simulink model "MDR_AA_TMD_Intercepteur"  (R2019b)
settings: Solver=ode4  StartTime=0.0  StopTime=Inf  FixedStep=0.01  RelTol=1e-3
values from neighbouring files (symbols this model uses):
  stdatm = [0 100 200 300 400 500 600 700 800 900 1000 1100 ... (4305 elements, 861x5)]    [stdatm.mat]
undefined symbols (not defined in the file or in its folder): Aero_Struct_CM, Aero_TMD, e0_0, e1_0, e2_0, e3_0, magnitude, Masse_Inertie_TMD, pow, Propu_TMD, Simu_TMD, Vm_0, xme_0
libraries: simulink x17
(part 4 of 4)

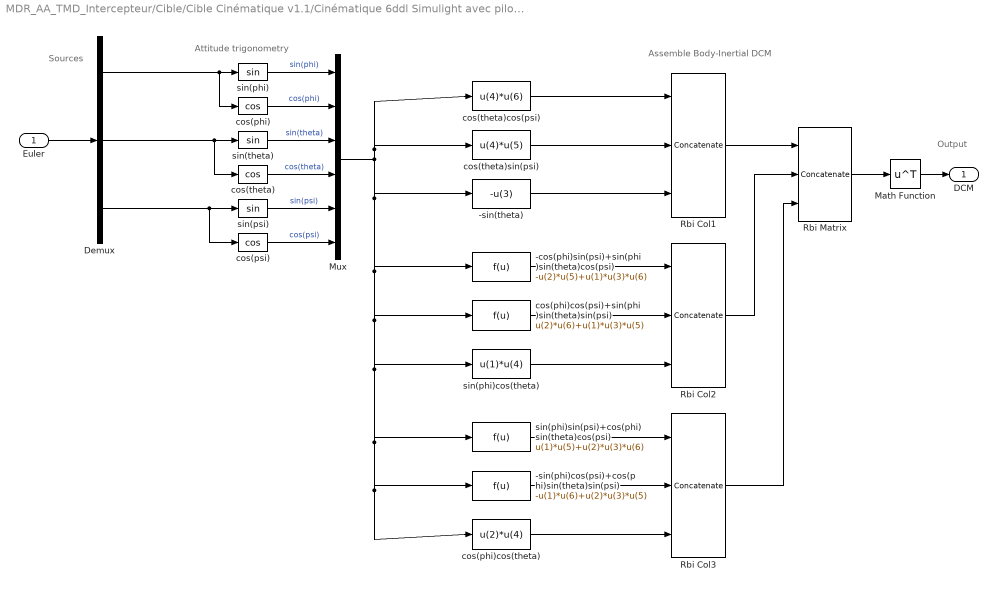
== system MDR_AA_TMD_Intercepteur/Cible/Cible Cinématique v1.1/Cinématique 6ddl Simulight avec pilotage en force/Pesanteur/Inert2Miss/Euler2DCM ==
  note: Attitude trigonometry
  note: Sources
  note: Output
  note: Assemble Body-Inertial DCM
  Euler : Inport  PortDimensions=[3 1]
  -cos(phi)sin(psi)+sin(phi)sin(theta)cos(psi) : Fcn  Expr=-u(2)*u(5)+u(1)*u(3)*u(6)
  -sin(phi)cos(psi)+cos(phi)sin(theta)sin(psi) : Fcn  Expr=-u(1)*u(6)+u(2)*u(3)*u(5)
  -sin(theta) : Fcn  Expr=-u(3)
  Demux : Demux  Outputs=3
  Math Function : Math  Operator=transpose  SaturateOnIntegerOverflow=on
  Mux : Mux  Inputs=6
  Rbi Matrix : Concatenate  NumInputs=3  Mode=Multidimensional array  ConcatenateDimension=2
  Rbi Col1 : Concatenate  NumInputs=3  Mode=Multidimensional array
  Rbi Col2 : Concatenate  NumInputs=3  Mode=Multidimensional array
  Rbi Col3 : Concatenate  NumInputs=3  Mode=Multidimensional array
  cos(phi) : Trigonometry  Operator=cos
  cos(phi)cos(psi)+sin(phi)sin(theta)sin(psi) : Fcn  Expr=u(2)*u(6)+u(1)*u(3)*u(5)
  cos(phi)cos(theta) : Fcn  Expr=u(2)*u(4)
  cos(psi) : Trigonometry  Operator=cos
  cos(theta) : Trigonometry  Operator=cos
  cos(theta)cos(psi) : Fcn  Expr=u(4)*u(6)
  cos(theta)sin(psi) : Fcn  Expr=u(4)*u(5)
  sin(phi) : Trigonometry
  sin(phi)cos(theta) : Fcn  Expr=u(1)*u(4)
  sin(phi)sin(psi)+cos(phi)sin(theta)cos(psi) : Fcn  Expr=u(1)*u(5)+u(2)*u(3)*u(6)
  sin(psi) : Trigonometry
  sin(theta) : Trigonometry
  DCM : Outport  VectorParamsAs1DForOutWhenUnconnected=off
  wires:
  Demux/3 -> sin(psi)/1, cos(psi)/1
  Demux/2 -> sin(theta)/1, cos(theta)/1
  Demux/1 -> cos(phi)/1, sin(phi)/1
  Euler/1 -> Demux/1
  sin(phi)/1 -> Mux/1  "sin(phi)"
  cos(phi)/1 -> Mux/2  "cos(phi)"
  sin(theta)/1 -> Mux/3  "sin(theta)"
  cos(theta)/1 -> Mux/4  "cos(theta)"
  sin(psi)/1 -> Mux/5  "sin(psi)"
  cos(psi)/1 -> Mux/6  "cos(psi)"
  Mux/1 -> cos(theta)cos(psi)/1, cos(theta)sin(psi)/1, sin(phi)sin(psi)+cos(phi)sin(theta)cos(psi)/1, cos(phi)cos(theta)/1, -sin(phi)cos(psi)+cos(phi)sin(theta)sin(psi)/1, sin(phi)cos(theta)/1, cos(phi)cos(psi)+sin(phi)sin(theta)sin(psi)/1, -cos(phi)sin(psi)+sin(phi)sin(theta)cos(psi)/1, -sin(theta)/1
  Math Function/1 -> DCM/1
  Rbi Matrix/1 -> Math Function/1
  Rbi Col1/1 -> Rbi Matrix/1
  cos(theta)cos(psi)/1 -> Rbi Col1/1
  cos(theta)sin(psi)/1 -> Rbi Col1/2
  -sin(theta)/1 -> Rbi Col1/3
  -cos(phi)sin(psi)+sin(phi)sin(theta)cos(psi)/1 -> Rbi Col2/1
  cos(phi)cos(psi)+sin(phi)sin(theta)sin(psi)/1 -> Rbi Col2/2
  sin(phi)cos(theta)/1 -> Rbi Col2/3
  sin(phi)sin(psi)+cos(phi)sin(theta)cos(psi)/1 -> Rbi Col3/1
  -sin(phi)cos(psi)+cos(phi)sin(theta)sin(psi)/1 -> Rbi Col3/2
  cos(phi)cos(theta)/1 -> Rbi Col3/3
  Rbi Col2/1 -> Rbi Matrix/2
  Rbi Col3/1 -> Rbi Matrix/3

== system MDR_AA_TMD_Intercepteur/Cible/Cible Cinématique v1.1/Pilote 2 axes Simulight à partir de gradient/Alpha commandé - Plan de tangage/Zero Offset/Non-zero Sign ==
  In : Inport
  One : Constant
  Relational Operator : RelationalOperator  Operator===  RndMeth=Nearest  InputSameDT=on
  Sign : Signum
  Switch : Switch  Threshold=1  SaturateOnIntegerOverflow=on  InputSameDT=on
  Zero : Constant  Value=0
  Out : Outport  VectorParamsAs1DForOutWhenUnconnected=off
  wires:
  Switch/1 -> Out/1
  Sign/1 -> Switch/3
  One/1 -> Switch/1
  Relational Operator/1 -> Switch/2
  In/1 -> Sign/1, Relational Operator/1
  Zero/1 -> Relational Operator/2

== system MDR_AA_TMD_Intercepteur/Cible/Cible Cinématique v1.1/Pilote 2 axes Simulight à partir de gradient/Beta commandé - Plan de lacet/Zero Offset/Non-zero Sign ==
  In : Inport
  One : Constant
  Relational Operator : RelationalOperator  Operator===  RndMeth=Nearest  InputSameDT=on
  Sign : Signum
  Switch : Switch  Threshold=1  SaturateOnIntegerOverflow=on  InputSameDT=on
  Zero : Constant  Value=0
  Out : Outport  VectorParamsAs1DForOutWhenUnconnected=off
  wires:
  Zero/1 -> Relational Operator/2
  In/1 -> Relational Operator/1, Sign/1
  Relational Operator/1 -> Switch/2
  One/1 -> Switch/1
  Sign/1 -> Switch/3
  Switch/1 -> Out/1

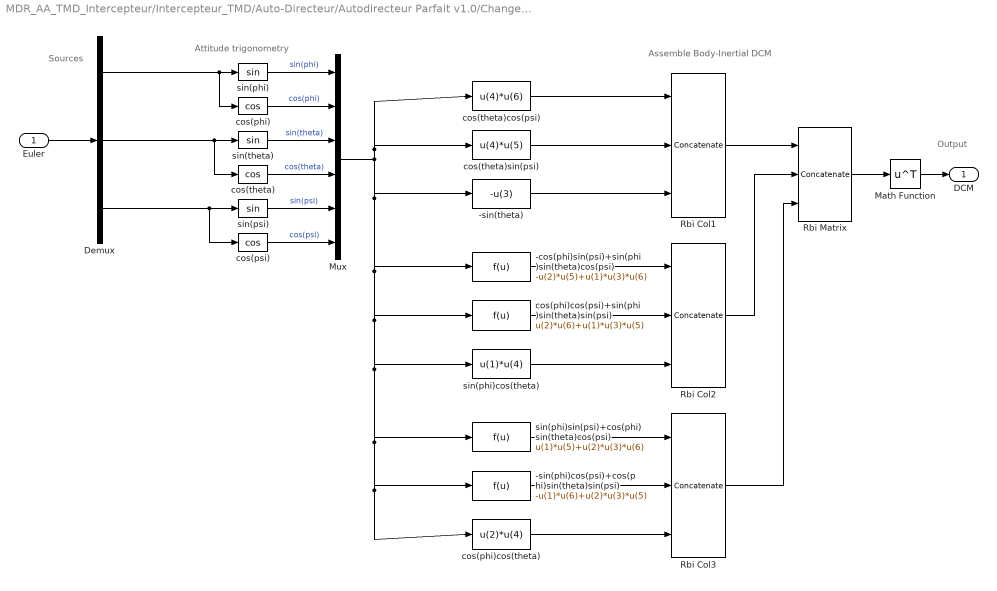
== system MDR_AA_TMD_Intercepteur/Intercepteur_TMD/Auto-Directeur/Autodirecteur Parfait v1.0/Changement de repère inertiel -> miss/Inert2Miss1/Euler2DCM ==
  note: Attitude trigonometry
  note: Sources
  note: Output
  note: Assemble Body-Inertial DCM
  Euler : Inport  PortDimensions=[3 1]
  -cos(phi)sin(psi)+sin(phi)sin(theta)cos(psi) : Fcn  Expr=-u(2)*u(5)+u(1)*u(3)*u(6)
  -sin(phi)cos(psi)+cos(phi)sin(theta)sin(psi) : Fcn  Expr=-u(1)*u(6)+u(2)*u(3)*u(5)
  -sin(theta) : Fcn  Expr=-u(3)
  Demux : Demux  Outputs=3
  Math Function : Math  Operator=transpose  SaturateOnIntegerOverflow=on
  Mux : Mux  Inputs=6
  Rbi Matrix : Concatenate  NumInputs=3  Mode=Multidimensional array  ConcatenateDimension=2
  Rbi Col1 : Concatenate  NumInputs=3  Mode=Multidimensional array
  Rbi Col2 : Concatenate  NumInputs=3  Mode=Multidimensional array
  Rbi Col3 : Concatenate  NumInputs=3  Mode=Multidimensional array
  cos(phi) : Trigonometry  Operator=cos
  cos(phi)cos(psi)+sin(phi)sin(theta)sin(psi) : Fcn  Expr=u(2)*u(6)+u(1)*u(3)*u(5)
  cos(phi)cos(theta) : Fcn  Expr=u(2)*u(4)
  cos(psi) : Trigonometry  Operator=cos
  cos(theta) : Trigonometry  Operator=cos
  cos(theta)cos(psi) : Fcn  Expr=u(4)*u(6)
  cos(theta)sin(psi) : Fcn  Expr=u(4)*u(5)
  sin(phi) : Trigonometry
  sin(phi)cos(theta) : Fcn  Expr=u(1)*u(4)
  sin(phi)sin(psi)+cos(phi)sin(theta)cos(psi) : Fcn  Expr=u(1)*u(5)+u(2)*u(3)*u(6)
  sin(psi) : Trigonometry
  sin(theta) : Trigonometry
  DCM : Outport  VectorParamsAs1DForOutWhenUnconnected=off
  wires:
  Demux/3 -> sin(psi)/1, cos(psi)/1
  Demux/2 -> sin(theta)/1, cos(theta)/1
  Demux/1 -> cos(phi)/1, sin(phi)/1
  Euler/1 -> Demux/1
  sin(phi)/1 -> Mux/1  "sin(phi)"
  cos(phi)/1 -> Mux/2  "cos(phi)"
  sin(theta)/1 -> Mux/3  "sin(theta)"
  cos(theta)/1 -> Mux/4  "cos(theta)"
  sin(psi)/1 -> Mux/5  "sin(psi)"
  cos(psi)/1 -> Mux/6  "cos(psi)"
  Mux/1 -> cos(theta)cos(psi)/1, cos(theta)sin(psi)/1, sin(phi)sin(psi)+cos(phi)sin(theta)cos(psi)/1, cos(phi)cos(theta)/1, -sin(phi)cos(psi)+cos(phi)sin(theta)sin(psi)/1, sin(phi)cos(theta)/1, cos(phi)cos(psi)+sin(phi)sin(theta)sin(psi)/1, -cos(phi)sin(psi)+sin(phi)sin(theta)cos(psi)/1, -sin(theta)/1
  Math Function/1 -> DCM/1
  Rbi Matrix/1 -> Math Function/1
  Rbi Col1/1 -> Rbi Matrix/1
  cos(theta)cos(psi)/1 -> Rbi Col1/1
  cos(theta)sin(psi)/1 -> Rbi Col1/2
  -sin(theta)/1 -> Rbi Col1/3
  -cos(phi)sin(psi)+sin(phi)sin(theta)cos(psi)/1 -> Rbi Col2/1
  cos(phi)cos(psi)+sin(phi)sin(theta)sin(psi)/1 -> Rbi Col2/2
  sin(phi)cos(theta)/1 -> Rbi Col2/3
  sin(phi)sin(psi)+cos(phi)sin(theta)cos(psi)/1 -> Rbi Col3/1
  -sin(phi)cos(psi)+cos(phi)sin(theta)sin(psi)/1 -> Rbi Col3/2
  cos(phi)cos(theta)/1 -> Rbi Col3/3
  Rbi Col2/1 -> Rbi Matrix/2
  Rbi Col3/1 -> Rbi Matrix/3

== system MDR_AA_TMD_Intercepteur/Intercepteur_TMD/Bloc Cinématique/Cinématique 6ddl Simulight avec pilotage en force/Calcul des pqr/pqr_a/dérive alpha//beta ==
  AlphaR : Inport
  BetaR : Inport  Port=2
  Clock : Clock
  Divide : Product  Inputs=*/
  Divide1 : Product  Inputs=*/
  IC : InitialCondition
  Memory : Memory
  Memory1 : Memory
  Memory2 : Memory
  Sum : Sum  Inputs=|+-
  Sum1 : Sum  Inputs=|+-
  Sum2 : Sum  Inputs=|+-
  dAlphaR : Outport  VectorParamsAs1DForOutWhenUnconnected=off
  dBetaR : Outport  Port=2  VectorParamsAs1DForOutWhenUnconnected=off
  wires:
  AlphaR/1 -> Memory/1, Sum/1
  Memory/1 -> Sum/2
  Sum/1 -> Divide/1
  BetaR/1 -> Sum1/1, Memory1/1
  Memory1/1 -> Sum1/2
  Sum1/1 -> Divide1/1
  Divide/1 -> dAlphaR/1
  Divide1/1 -> dBetaR/1
  Clock/1 -> Memory2/1, Sum2/1
  Memory2/1 -> Sum2/2
  Sum2/1 -> IC/1
  IC/1 -> Divide1/2, Divide/2

== system MDR_AA_TMD_Intercepteur/Intercepteur_TMD/Bloc Cinématique/Cinématique 6ddl Simulight avec pilotage en force/Equations des forces/Gestion de sortie de rampe/Norme ==
  V : Inport
  Dot Product : DotProduct  InputSameDT=on  OutDataTypeStr=Inherit: Inherit via internal rule
  Sqrt : Math  Operator=sqrt  SaturateOnIntegerOverflow=on
  ||V|| : Outport  VectorParamsAs1DForOutWhenUnconnected=off
  wires:
  Sqrt/1 -> ||V||/1
  V/1 -> Dot Product/2, Dot Product/1
  Dot Product/1 -> Sqrt/1

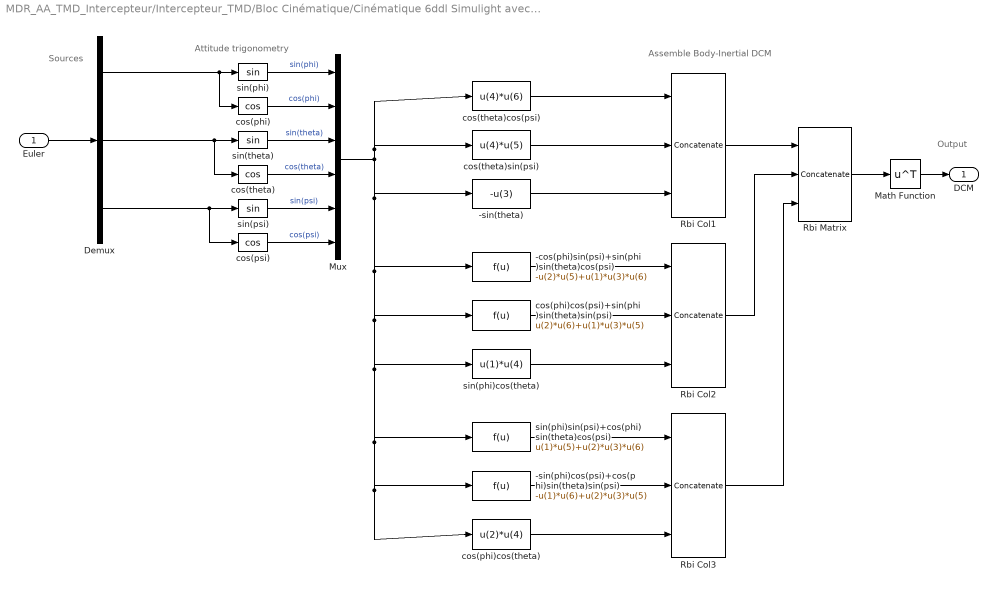
== system MDR_AA_TMD_Intercepteur/Intercepteur_TMD/Bloc Cinématique/Cinématique 6ddl Simulight avec pilotage en force/Pesanteur/Inert2Miss/Euler2DCM ==
  note: Attitude trigonometry
  note: Sources
  note: Output
  note: Assemble Body-Inertial DCM
  Euler : Inport  PortDimensions=[3 1]
  -cos(phi)sin(psi)+sin(phi)sin(theta)cos(psi) : Fcn  Expr=-u(2)*u(5)+u(1)*u(3)*u(6)
  -sin(phi)cos(psi)+cos(phi)sin(theta)sin(psi) : Fcn  Expr=-u(1)*u(6)+u(2)*u(3)*u(5)
  -sin(theta) : Fcn  Expr=-u(3)
  Demux : Demux  Outputs=3
  Math Function : Math  Operator=transpose  SaturateOnIntegerOverflow=on
  Mux : Mux  Inputs=6
  Rbi Matrix : Concatenate  NumInputs=3  Mode=Multidimensional array  ConcatenateDimension=2
  Rbi Col1 : Concatenate  NumInputs=3  Mode=Multidimensional array
  Rbi Col2 : Concatenate  NumInputs=3  Mode=Multidimensional array
  Rbi Col3 : Concatenate  NumInputs=3  Mode=Multidimensional array
  cos(phi) : Trigonometry  Operator=cos
  cos(phi)cos(psi)+sin(phi)sin(theta)sin(psi) : Fcn  Expr=u(2)*u(6)+u(1)*u(3)*u(5)
  cos(phi)cos(theta) : Fcn  Expr=u(2)*u(4)
  cos(psi) : Trigonometry  Operator=cos
  cos(theta) : Trigonometry  Operator=cos
  cos(theta)cos(psi) : Fcn  Expr=u(4)*u(6)
  cos(theta)sin(psi) : Fcn  Expr=u(4)*u(5)
  sin(phi) : Trigonometry
  sin(phi)cos(theta) : Fcn  Expr=u(1)*u(4)
  sin(phi)sin(psi)+cos(phi)sin(theta)cos(psi) : Fcn  Expr=u(1)*u(5)+u(2)*u(3)*u(6)
  sin(psi) : Trigonometry
  sin(theta) : Trigonometry
  DCM : Outport  VectorParamsAs1DForOutWhenUnconnected=off
  wires:
  Demux/3 -> sin(psi)/1, cos(psi)/1
  Demux/2 -> sin(theta)/1, cos(theta)/1
  Demux/1 -> cos(phi)/1, sin(phi)/1
  Euler/1 -> Demux/1
  sin(phi)/1 -> Mux/1  "sin(phi)"
  cos(phi)/1 -> Mux/2  "cos(phi)"
  sin(theta)/1 -> Mux/3  "sin(theta)"
  cos(theta)/1 -> Mux/4  "cos(theta)"
  sin(psi)/1 -> Mux/5  "sin(psi)"
  cos(psi)/1 -> Mux/6  "cos(psi)"
  Mux/1 -> cos(theta)cos(psi)/1, cos(theta)sin(psi)/1, sin(phi)sin(psi)+cos(phi)sin(theta)cos(psi)/1, cos(phi)cos(theta)/1, -sin(phi)cos(psi)+cos(phi)sin(theta)sin(psi)/1, sin(phi)cos(theta)/1, cos(phi)cos(psi)+sin(phi)sin(theta)sin(psi)/1, -cos(phi)sin(psi)+sin(phi)sin(theta)cos(psi)/1, -sin(theta)/1
  Math Function/1 -> DCM/1
  Rbi Matrix/1 -> Math Function/1
  Rbi Col1/1 -> Rbi Matrix/1
  cos(theta)cos(psi)/1 -> Rbi Col1/1
  cos(theta)sin(psi)/1 -> Rbi Col1/2
  -sin(theta)/1 -> Rbi Col1/3
  -cos(phi)sin(psi)+sin(phi)sin(theta)cos(psi)/1 -> Rbi Col2/1
  cos(phi)cos(psi)+sin(phi)sin(theta)sin(psi)/1 -> Rbi Col2/2
  sin(phi)cos(theta)/1 -> Rbi Col2/3
  sin(phi)sin(psi)+cos(phi)sin(theta)cos(psi)/1 -> Rbi Col3/1
  -sin(phi)cos(psi)+cos(phi)sin(theta)sin(psi)/1 -> Rbi Col3/2
  cos(phi)cos(theta)/1 -> Rbi Col3/3
  Rbi Col2/1 -> Rbi Matrix/2
  Rbi Col3/1 -> Rbi Matrix/3

== system MDR_AA_TMD_Intercepteur/Intercepteur_TMD/Calculateur/Pilotage/Pilote 2 axes Simulight avec prise en compte de la manoeuvrabilité max/Alpha commandé - Plan de tangage/Calcul de CN0 ==
  Alpha : Inport
  Mach : Inport  Port=2
  CN_0 : Lookup_n-D  BreakpointsForDimension1=vAlpha  BreakpointsForDimension2=vMach  BreakpointsForDimension3=Aero_Struct_CM.vBrq  Table=CN  ExtrapMethod=Clip  UseLastTableValue=on  RndMeth=Simplest  InputSameDT=on
  vCN0 : Outport  VectorParamsAs1DForOutWhenUnconnected=off
  wires:
  CN_0/1 -> vCN0/1
  Mach/1 -> CN_0/2
  Alpha/1 -> CN_0/1

== system MDR_AA_TMD_Intercepteur/Intercepteur_TMD/Calculateur/Pilotage/Pilote 2 axes Simulight avec prise en compte de la manoeuvrabilité max/Alpha commandé - Plan de tangage/Calcul du coefficient de CN commandé avec gestion de la division par 0 ==
  GcoV : Inport
  Masse : Inport  Port=2
  Pression_dynamique : Inport  Port=3
  Compare To Zero : simulink/Logic and Bit Operations/Compare To Zero  relop===  OutDataTypeStr=boolean  ZeroCross=off
  Divide1 : Product  Inputs=*/
  Memory : Memory
  Product : Product  RndMeth=Zero
  Switch : Switch  Criteria=u2 > Threshold
  Zero Offset : Subsystem  mask(Zero offset){tol=10^-6}
      mask prompts: tol "Tolerance"
      mask help: This block outputs a value equal to the tolerance specified in the block parameters if the input falls within a sphere with this tolerance as radius and center in the origin. Otherwise, the output equals the input.
      mask Help: eval('OpenHelp(''A3_Blockset.mdl'', ''..\Help\Toolbox\Tools\Zero_offset.html'')');
  CN_co : Outport  VectorParamsAs1DForOutWhenUnconnected=off
  wires:
  Pression_dynamique/1 -> Compare To Zero/1, Zero Offset/1(In)
  Switch/1 -> CN_co/1, Memory/1
  Compare To Zero/1 -> Switch/2
  GcoV/1 -> Product/2
  Masse/1 -> Divide1/1
  Divide1/1 -> Product/1
  Product/1 -> Switch/3
  Memory/1 -> Switch/1
  Zero Offset/1(Out) -> Divide1/2

== system MDR_AA_TMD_Intercepteur/Intercepteur_TMD/Calculateur/Pilotage/Pilote 2 axes Simulight avec prise en compte de la manoeuvrabilité max/Alpha commandé - Plan de tangage/Interpolation linéaire pour trouver l'incidence correspondant au coefficient de portance commandé ==
  CN_co_sat : Inport
  vCN0 : Inport  Port=2
  vAlpha : Inport  Port=3
  Lookup Table Dynamic : simulink/Lookup Tables/Lookup Table Dynamic  LookUpMeth=Interpolation-Use End Values  OutDataType=fixdt('double')  OutScaling=[]  OutputDataTypeScalingMode=Specify via dialog  OutDataTypeStr=fixdt('double')  DoSatur=off
      settings: SourceProductName=Simulink
  deg2rad : Gain  Gain=pi/180
  Alphaco : Outport  VectorParamsAs1DForOutWhenUnconnected=off
  wires:
  deg2rad/1 -> Alphaco/1
  vCN0/1 -> Lookup Table Dynamic/2
  CN_co_sat/1 -> Lookup Table Dynamic/1
  vAlpha/1 -> Lookup Table Dynamic/3
  Lookup Table Dynamic/1 -> deg2rad/1

== system MDR_AA_TMD_Intercepteur/Intercepteur_TMD/Calculateur/Pilotage/Pilote 2 axes Simulight avec prise en compte de la manoeuvrabilité max/Alpha commandé - Plan de tangage/Saturation de CN_co par la valeur max de CN équilibré ==
  Mach : Inport
  CN_co : Inport  Port=2
  CNmax : Lookup_n-D  NumberOfTableDimensions=1  BreakpointsForDimension1=vMach_CNmax  Table=CNmax  ExtrapMethod=Clip  UseLastTableValue=on  RndMeth=Simplest  InputSameDT=on
  Gain : Gain  Gain=-1
  Saturation Dynamic : simulink/Discontinuities/Saturation Dynamic  OutMin=[]  OutMax=[]  OutDataTypeStr=Inherit: Same as second input  OutDataType=fixdt(1, 16)  OutScaling=2^-10  DoSatur=off
  CN_co_sat : Outport  VectorParamsAs1DForOutWhenUnconnected=off
  wires:
  Saturation Dynamic/1 -> CN_co_sat/1
  CN_co/1 -> Saturation Dynamic/2
  Mach/1 -> CNmax/1
  Gain/1 -> Saturation Dynamic/3
  CNmax/1 -> Gain/1, Saturation Dynamic/1

== system MDR_AA_TMD_Intercepteur/Intercepteur_TMD/Calculateur/Pilotage/Pilote 2 axes Simulight avec prise en compte de la manoeuvrabilité max/Beta commandé - Plan de lacet/Calcul de CY0 ==
  Beta : Inport
  Mach : Inport  Port=2
  CY_0 : Lookup_n-D  BreakpointsForDimension1=vBeta  BreakpointsForDimension2=vMach  BreakpointsForDimension3=Aero_Struct_CM.vBrq  Table=CY  ExtrapMethod=Clip  UseLastTableValue=on  RndMeth=Simplest  InputSameDT=on
  vCY0 : Outport  VectorParamsAs1DForOutWhenUnconnected=off
  wires:
  Beta/1 -> CY_0/1
  Mach/1 -> CY_0/2
  CY_0/1 -> vCY0/1

== system MDR_AA_TMD_Intercepteur/Intercepteur_TMD/Calculateur/Pilotage/Pilote 2 axes Simulight avec prise en compte de la manoeuvrabilité max/Beta commandé - Plan de lacet/Calcul du coefficient de CY commandé avec gestion de la division par 0 ==
  GcoH : Inport
  Masse : Inport  Port=2
  Pression_dynamique : Inport  Port=3
  Compare To Zero : simulink/Logic and Bit Operations/Compare To Zero  relop===  OutDataTypeStr=boolean  ZeroCross=off
  Divide1 : Product  Inputs=*/
  Memory : Memory
  Product : Product  RndMeth=Zero
  Switch : Switch  Criteria=u2 > Threshold
  Zero Offset : Subsystem  mask(Zero offset){tol=10^-6}
      mask prompts: tol "Tolerance"
      mask help: This block outputs a value equal to the tolerance specified in the block parameters if the input falls within a sphere with this tolerance as radius and center in the origin. Otherwise, the output equals the input.
      mask Help: eval('OpenHelp(''A3_Blockset.mdl'', ''..\Help\Toolbox\Tools\Zero_offset.html'')');
  CY_co : Outport  VectorParamsAs1DForOutWhenUnconnected=off
  wires:
  Pression_dynamique/1 -> Compare To Zero/1, Zero Offset/1(In)
  Switch/1 -> CY_co/1, Memory/1
  Compare To Zero/1 -> Switch/2
  GcoH/1 -> Product/2
  Masse/1 -> Divide1/1
  Divide1/1 -> Product/1
  Product/1 -> Switch/3
  Memory/1 -> Switch/1
  Zero Offset/1(Out) -> Divide1/2

== system MDR_AA_TMD_Intercepteur/Intercepteur_TMD/Calculateur/Pilotage/Pilote 2 axes Simulight avec prise en compte de la manoeuvrabilité max/Beta commandé - Plan de lacet/Interpolation linéaire pour trouver le dérapage correspondant au coefficient de portance commandé ==
  CY_co_sat : Inport
  vCY0 : Inport  Port=2
  vBeta : Inport  Port=3
  Lookup Table Dynamic : simulink/Lookup Tables/Lookup Table Dynamic  LookUpMeth=Interpolation-Use End Values  OutDataType=fixdt('double')  OutScaling=[]  OutputDataTypeScalingMode=Specify via dialog  OutDataTypeStr=fixdt('double')  DoSatur=off
      settings: SourceProductName=Simulink
  deg2rad : Gain  Gain=pi/180
  Betaco : Outport  VectorParamsAs1DForOutWhenUnconnected=off
  wires:
  Lookup Table Dynamic/1 -> deg2rad/1
  vBeta/1 -> Lookup Table Dynamic/3
  CY_co_sat/1 -> Lookup Table Dynamic/1
  vCY0/1 -> Lookup Table Dynamic/2
  deg2rad/1 -> Betaco/1

== system MDR_AA_TMD_Intercepteur/Intercepteur_TMD/Calculateur/Pilotage/Pilote 2 axes Simulight avec prise en compte de la manoeuvrabilité max/Beta commandé - Plan de lacet/Saturation de CN_co par la valeur max de CN équilibré ==
  Mach : Inport
  CY_co : Inport  Port=2
  CYmax : Lookup_n-D  NumberOfTableDimensions=1  BreakpointsForDimension1=vMach_CYmax  Table=CYmax  ExtrapMethod=Clip  UseLastTableValue=on  RndMeth=Simplest  InputSameDT=on
  Gain : Gain  Gain=-1
  Saturation Dynamic : simulink/Discontinuities/Saturation Dynamic  OutMin=[]  OutMax=[]  OutDataTypeStr=Inherit: Same as second input  OutDataType=fixdt(1, 16)  OutScaling=2^-10  DoSatur=off
  CY_co_sat : Outport  VectorParamsAs1DForOutWhenUnconnected=off
  wires:
  CYmax/1 -> Gain/1, Saturation Dynamic/1
  Gain/1 -> Saturation Dynamic/3
  Mach/1 -> CYmax/1
  CY_co/1 -> Saturation Dynamic/2
  Saturation Dynamic/1 -> CY_co_sat/1

== system MDR_AA_TMD_Intercepteur/Intercepteur_TMD/Calculateur/Pilotage/Pilote 2 axes Simulight avec prise en compte de la manoeuvrabilité max/Calcul du Mach/Norme ==
  V : Inport
  Dot Product : DotProduct  InputSameDT=on  OutDataTypeStr=Inherit: Inherit via internal rule
  Sqrt : Math  Operator=sqrt  SaturateOnIntegerOverflow=on
  ||V|| : Outport  VectorParamsAs1DForOutWhenUnconnected=off
  wires:
  Sqrt/1 -> ||V||/1
  V/1 -> Dot Product/2, Dot Product/1
  Dot Product/1 -> Sqrt/1

== system MDR_AA_TMD_Intercepteur/Intercepteur_TMD/Forces-Moments/Propulsion de l'exemple TMD/Propulsion Booster/Calcul de la force de poussée/Calcul de la force de poussée ==
  note: ( \pi D^2 ) / (4. 10^6)
  debit_propu : Inport
  g : Inport  Port=2
  Pression_statique : Inport  Port=3
  Action Port : ActionPort  PropagateVarSize=During execution
  Add : Sum  Inputs=-+
  Add1 : Sum
  Constant : Constant  Value=Booster_Isp  SampleTime=Inf
  Constant3 : Constant  Value=Diametre_tuy  SampleTime=Inf
  Gain2 : Gain  Gain=pi
  Gain3 : Gain  Gain=1/(4*10^6)
  Math Function1 : Math  Operator=magnitude^2  SaturateOnIntegerOverflow=on
  Pression au niveau du sol en Pa : Constant  Value=101325  SampleTime=Inf
  Product : Product  Inputs=3  RndMeth=Zero
  Product1 : Product  RndMeth=Zero
  Force_poussee : Outport  VectorParamsAs1DForOutWhenUnconnected=off
  wires:
  Math Function1/1 -> Product1/2
  Constant3/1 -> Math Function1/1
  Gain3/1 -> Add1/2
  Gain2/1 -> Gain3/1
  Product1/1 -> Gain2/1
  Constant/1 -> Product/3
  g/1 -> Product/2
  debit_propu/1 -> Product/1
  Pression_statique/1 -> Add/1
  Pression au niveau du sol en Pa/1 -> Add/2
  Add/1 -> Product1/1
  Product/1 -> Add1/1
  Add1/1 -> Force_poussee/1

== system MDR_AA_TMD_Intercepteur/Intercepteur_TMD/Forces-Moments/Propulsion de l'exemple TMD/Propulsion Booster/Calcul de la force de poussée/Sans force de poussee ==
  Action Port : ActionPort  PropagateVarSize=During execution
  Constant : Constant  Value=0  SampleTime=Inf
  Force_poussee : Outport  InitialOutput=0  VectorParamsAs1DForOutWhenUnconnected=off
  wires:
  Constant/1 -> Force_poussee/1

== system MDR_AA_TMD_Intercepteur/Intercepteur_TMD/Forces-Moments/Propulsion de l'exemple TMD/Propulsion Croisiere/Calcul de la force de poussée/Calcul de la force de poussée ==
  note: ( \pi D^2 ) / (4. 10^6)
  debit_propu : Inport
  g : Inport  Port=2
  Pression_statique : Inport  Port=3
  Action Port : ActionPort  PropagateVarSize=During execution
  Add : Sum  Inputs=-+
  Add1 : Sum
  Constant : Constant  Value=Booster_Isp  SampleTime=Inf
  Constant3 : Constant  Value=Diametre_tuy  SampleTime=Inf
  Gain2 : Gain  Gain=pi
  Gain3 : Gain  Gain=1/(4*10^6)
  Math Function1 : Math  Operator=magnitude^2  SaturateOnIntegerOverflow=on
  Pression au niveau du sol en Pa : Constant  Value=101325  SampleTime=Inf
  Product : Product  Inputs=3  RndMeth=Zero
  Product1 : Product  RndMeth=Zero
  Force_poussee : Outport  VectorParamsAs1DForOutWhenUnconnected=off
  wires:
  Math Function1/1 -> Product1/2
  Constant3/1 -> Math Function1/1
  Gain3/1 -> Add1/2
  Gain2/1 -> Gain3/1
  Product1/1 -> Gain2/1
  Constant/1 -> Product/3
  g/1 -> Product/2
  debit_propu/1 -> Product/1
  Pression_statique/1 -> Add/1
  Pression au niveau du sol en Pa/1 -> Add/2
  Add/1 -> Product1/1
  Product/1 -> Add1/1
  Add1/1 -> Force_poussee/1

== system MDR_AA_TMD_Intercepteur/Intercepteur_TMD/Forces-Moments/Propulsion de l'exemple TMD/Propulsion Croisiere/Calcul de la force de poussée/Sans force de poussee ==
  Action Port : ActionPort  PropagateVarSize=During execution
  Constant : Constant  Value=0  SampleTime=Inf
  Force_poussee : Outport  InitialOutput=0  VectorParamsAs1DForOutWhenUnconnected=off
  wires:
  Constant/1 -> Force_poussee/1

== system MDR_AA_TMD_Intercepteur/Modèle de terre/xyz_NED2LLA/ECEF2LLA/Calcul de la latitude/Calcul de mu/f ==
  (1-e^2) : Subsystem
  1 : Constant
  Sqrt : Sqrt  SaturateOnIntegerOverflow=on
  Subtract : Sum  Inputs=+-
  f : Outport  VectorParamsAs1DForOutWhenUnconnected=off
  wires:
  Sqrt/1 -> Subtract/2
  (1-e^2)/1((1-e^2)) -> Sqrt/1
  Subtract/1 -> f/1
  1/1 -> Subtract/1

== system MDR_AA_TMD_Intercepteur/Intercepteur_TMD/Calculateur/Pilotage/Pilote 2 axes Simulight avec prise en compte de la manoeuvrabilité max/Alpha commandé - Plan de tangage/Calcul du coefficient de CN commandé avec gestion de la division par 0/Zero Offset ==
  In : Inport
  Abs : Abs  SaturateOnIntegerOverflow=on
  Constant : Constant  Value=tol
  Non-zero Sign : Subsystem  mask(Non-zero sign){}
      mask help: Sign function outputs 1 for input greater than or equal to 0, and -1 otherwise.
  Product : Product  SaturateOnIntegerOverflow=on  RndMeth=Zero  InputSameDT=on  OutDataTypeStr=Inherit: Same as first input
  Switch : Switch  Threshold=tol  SaturateOnIntegerOverflow=on  InputSameDT=on
  Out : Outport  VectorParamsAs1DForOutWhenUnconnected=off
  wires:
  Switch/1 -> Out/1
  Product/1 -> Switch/3
  Constant/1 -> Product/2
  Non-zero Sign/1(Out) -> Product/1
  Abs/1 -> Switch/2
  In/1 -> Abs/1, Non-zero Sign/1(In), Switch/1

== system MDR_AA_TMD_Intercepteur/Intercepteur_TMD/Calculateur/Pilotage/Pilote 2 axes Simulight avec prise en compte de la manoeuvrabilité max/Beta commandé - Plan de lacet/Calcul du coefficient de CY commandé avec gestion de la division par 0/Zero Offset ==
  In : Inport
  Abs : Abs  SaturateOnIntegerOverflow=on
  Constant : Constant  Value=tol
  Non-zero Sign : Subsystem  mask(Non-zero sign){}
      mask help: Sign function outputs 1 for input greater than or equal to 0, and -1 otherwise.
  Product : Product  SaturateOnIntegerOverflow=on  RndMeth=Zero  InputSameDT=on  OutDataTypeStr=Inherit: Same as first input
  Switch : Switch  Threshold=tol  SaturateOnIntegerOverflow=on  InputSameDT=on
  Out : Outport  VectorParamsAs1DForOutWhenUnconnected=off
  wires:
  Switch/1 -> Out/1
  Product/1 -> Switch/3
  Constant/1 -> Product/2
  Non-zero Sign/1(Out) -> Product/1
  Abs/1 -> Switch/2
  In/1 -> Abs/1, Non-zero Sign/1(In), Switch/1

== system MDR_AA_TMD_Intercepteur/Modèle de terre/xyz_NED2LLA/ECEF2LLA/Calcul de la latitude/Calcul de mu/f/(1-e^2) ==
  Constant : Constant
  Math Function : Math  Operator=magnitude^2  SaturateOnIntegerOverflow=on
  Sum : Sum  Inputs=|+-
  e : Constant  Value=e
  (1-e^2) : Outport  VectorParamsAs1DForOutWhenUnconnected=off
  wires:
  Constant/1 -> Sum/1
  Math Function/1 -> Sum/2
  Sum/1 -> (1-e^2)/1
  e/1 -> Math Function/1

== system MDR_AA_TMD_Intercepteur/Intercepteur_TMD/Calculateur/Pilotage/Pilote 2 axes Simulight avec prise en compte de la manoeuvrabilité max/Alpha commandé - Plan de tangage/Calcul du coefficient de CN commandé avec gestion de la division par 0/Zero Offset/Non-zero Sign ==
  In : Inport
  One : Constant
  Relational Operator : RelationalOperator  Operator===  RndMeth=Nearest  InputSameDT=on
  Sign : Signum
  Switch : Switch  Threshold=1  SaturateOnIntegerOverflow=on  InputSameDT=on
  Zero : Constant  Value=0
  Out : Outport  VectorParamsAs1DForOutWhenUnconnected=off
  wires:
  Switch/1 -> Out/1
  Sign/1 -> Switch/3
  One/1 -> Switch/1
  Relational Operator/1 -> Switch/2
  In/1 -> Sign/1, Relational Operator/1
  Zero/1 -> Relational Operator/2

== system MDR_AA_TMD_Intercepteur/Intercepteur_TMD/Calculateur/Pilotage/Pilote 2 axes Simulight avec prise en compte de la manoeuvrabilité max/Beta commandé - Plan de lacet/Calcul du coefficient de CY commandé avec gestion de la division par 0/Zero Offset/Non-zero Sign ==
  In : Inport
  One : Constant
  Relational Operator : RelationalOperator  Operator===  RndMeth=Nearest  InputSameDT=on
  Sign : Signum
  Switch : Switch  Threshold=1  SaturateOnIntegerOverflow=on  InputSameDT=on
  Zero : Constant  Value=0
  Out : Outport  VectorParamsAs1DForOutWhenUnconnected=off
  wires:
  Switch/1 -> Out/1
  Sign/1 -> Switch/3
  One/1 -> Switch/1
  Relational Operator/1 -> Switch/2
  In/1 -> Sign/1, Relational Operator/1
  Zero/1 -> Relational Operator/2
